simulink model "Nivel_Concentracao_MF"  (R2020a)
settings: Solver=VariableStepAuto  StartTime=0.0  StopTime=40  RelTol=1e-3
libraries: cstblocks x18
settings Model: Creator=Avell  LastModifiedBy=Avell

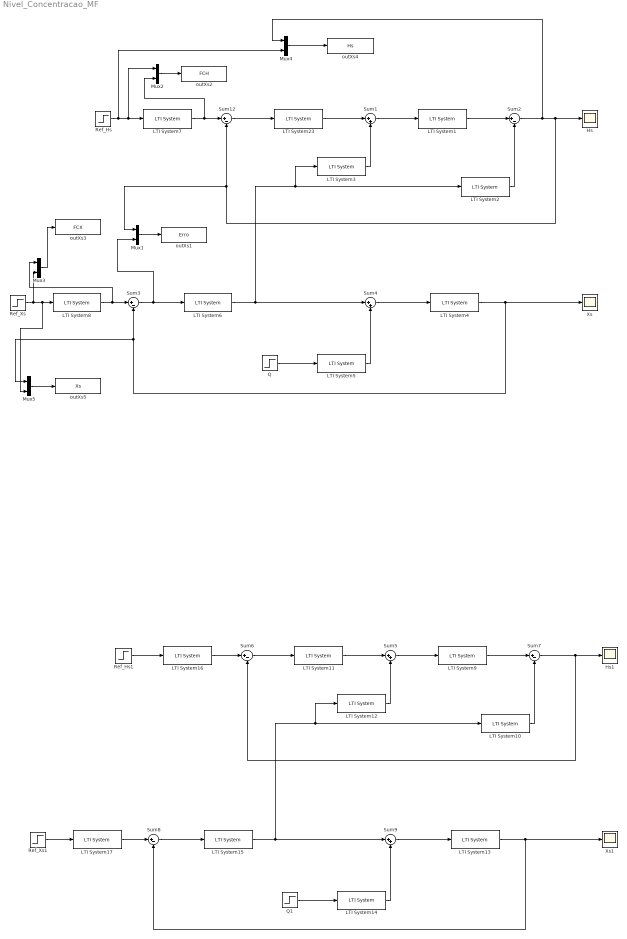
== system Nivel_Concentracao_MF ==
  Hs : Scope
  Hs1 : Scope
  LTI System1 : cstblocks/LTI System  sys=Gh  IC=[]
  LTI System10 : cstblocks/LTI System  sys=Gvc  IC=[]
  LTI System11 : cstblocks/LTI System  sys=CH  IC=[]
  LTI System12 : cstblocks/LTI System  sys=CffV  IC=[]
  LTI System13 : cstblocks/LTI System  sys=Gx  IC=[]
  LTI System14 : cstblocks/LTI System  sys=0.5  IC=[]
  LTI System15 : cstblocks/LTI System  sys=CX  IC=[]
  LTI System16 : cstblocks/LTI System  sys=FCH  IC=[]
  LTI System17 : cstblocks/LTI System  sys=FCX  IC=[]
  LTI System2 : cstblocks/LTI System  sys=Gvc  IC=[]
  LTI System23 : cstblocks/LTI System  sys=CH  IC=[]
  LTI System3 : cstblocks/LTI System  sys=CffV  IC=[]
  LTI System4 : cstblocks/LTI System  sys=Gx  IC=[]
  LTI System5 : cstblocks/LTI System  sys=0.5  IC=[]
  LTI System6 : cstblocks/LTI System  sys=CX  IC=[]
  LTI System7 : cstblocks/LTI System  sys=FCH  IC=[]
  LTI System8 : cstblocks/LTI System  sys=FCX  IC=[]
  LTI System9 : cstblocks/LTI System  sys=Gh  IC=[]
  Mux{1..5} (5 alike) : Mux  Inputs=2
  Q : Step  Time=20  SampleTime=0
  Q1 : Step  Time=20  SampleTime=0
  Ref_Hs : Step  Time=5  SampleTime=0
  Ref_Hs1 : Step  Time=5  SampleTime=0
  Ref_Xs : Step  Time=10  SampleTime=0
  Ref_Xs1 : Step  Time=10  SampleTime=0
  Sum{1,4..5,9} (4 alike) : Sum  Inputs=|++
  Sum{2..3,6..8,12} (6 alike) : Sum  Inputs=|+-
  Xs : Scope
  Xs1 : Scope
  outXs1 : ToWorkspace  VariableName=Erro  SaveFormat=Structure With Time  SampleTime=-1
  outXs2 : ToWorkspace  VariableName=FCH  SaveFormat=Structure With Time  SampleTime=-1
  outXs3 : ToWorkspace  VariableName=FCX  SaveFormat=Structure With Time  SampleTime=-1
  outXs4 : ToWorkspace  VariableName=Hs  SaveFormat=Structure With Time  SampleTime=-1
  outXs5 : ToWorkspace  VariableName=Xs  SaveFormat=Structure With Time  SampleTime=-1
  wires:
  LTI System23/1 -> Sum1/1
  Sum12/1 -> LTI System23/1
  Sum1/1 -> LTI System1/1
  LTI System1/1 -> Sum2/1
  LTI System2/1 -> Sum2/2
  Sum2/1 -> Mux4/1, Mux1/1, Sum12/2, Hs/1
  LTI System3/1 -> Sum1/2
  LTI System6/1 -> Sum4/1, LTI System3/1, LTI System2/1
  LTI System5/1 -> Sum4/2
  Sum3/1 -> Mux1/2, LTI System6/1
  Q/1 -> LTI System5/1
  LTI System7/1 -> Mux2/2, Sum12/1
  Ref_Hs/1 -> Mux4/2, Mux2/1, LTI System7/1
  LTI System8/1 -> Mux3/1, Sum3/1
  LTI System4/1 -> Xs/1, Mux5/1, Sum3/2
  Sum4/1 -> LTI System4/1
  Mux1/1 -> outXs1/1
  Mux2/1 -> outXs2/1
  Mux3/1 -> outXs3/1
  Ref_Xs/1 -> Mux3/2, Mux5/2, LTI System8/1
  Mux4/1 -> outXs4/1
  Mux5/1 -> outXs5/1
  LTI System13/1 -> Xs1/1, Sum8/2
  Sum6/1 -> LTI System11/1
  Sum9/1 -> LTI System13/1
  Sum5/1 -> LTI System9/1
  LTI System14/1 -> Sum9/2
  Ref_Xs1/1 -> LTI System17/1
  Sum8/1 -> LTI System15/1
  LTI System12/1 -> Sum5/2
  LTI System11/1 -> Sum5/1
  LTI System17/1 -> Sum8/1
  Ref_Hs1/1 -> LTI System16/1
  LTI System15/1 -> Sum9/1, LTI System12/1, LTI System10/1
  Q1/1 -> LTI System14/1
  LTI System10/1 -> Sum7/2
  Sum7/1 -> Sum6/2, Hs1/1
  LTI System16/1 -> Sum6/1
  LTI System9/1 -> Sum7/1
